simulink library "lib_fuel_converter"  (Simulink 4.00)
undefined symbols (not defined in the file): acc_mech_eff, acc_mech_pwr, acc_mech_trq, air_cp, amb_tmp, cyc_mph, ex_gas_cp, fc_acc_mass, fc_base_mass, fc_c2i_th_cond, fc_c_init_tmp, fc_cl2h_eff, fc_CO2_to_FUELgps, fc_cold, fc_cold_tmp, fc_cp, fc_ct_trq, fc_emisv, fc_ext_sarea, fc_fuel_den, fc_fuel_lhv, fc_h2x_th_cond, fc_h_air_flow, fc_h_cp, fc_h_init_tmp, fc_hood_emisv, fc_hood_sarea, fc_i2x_th_cond, fc_i_init_tmp, fc_inertia, fc_map_spd, fc_map_trq, fc_max_trq, fc_nn_model_name, fc_pwr_scale, fc_spd_scale, fc_trq_scale, fc_tstat, fc_x_init_tmp, fd_ratio, gb_num_init, gb_ratio, pow, vc_idle_spd, vc_key_on, veh_glider_mass, veh_mass, wh_radius
libraries: lib_fuel_converter x6, lib_etc x4
(part 1 of 4)
settings Model: Creator=NREL  LastModifiedBy=abrooker  ModifiedComment=abrooker -- Wed Jun 19 09:43:22 2002 -- Version 3.0440
settings Model: ModifiedHistory=|
  | abrooker -- Wed Jun 19 09:43:22 2002 -- Version 3.0440
  | 
  | 
  | abrooker -- Thu May 02 16:55:00 2002 -- Version 3.0439
  | deleted obsolete saber fc's
  | 
  | mokeefe -- Wed May 01 08:51:04 2002 -- Version 3.0438
  | changed the way scaling occurs on the FC temperature correction in the EO emissions and fuel usage block
  | 
  | tmarkel -- Tue Apr 30 08:52:52 2002 -- Version 3.0437
  | removed fuel cell model - moved to lib_fuel_cell
  | 
  | 
  | kharalds -- Thu Apr 25 16:04:02 2002 -- Version 3.0436
  | Removed the 4th input to Multi-port switches 1, 2, 3, 4 & blank (no number).
  | 
  | kharalds -- Fri Apr 19 16:04:21 2002 -- Version 3.0435
  | Removed fuel cell model option # 4 and its connections.
  | 
  | kharalds -- Fri Apr 19 08:05:59 2002 -- Version 3.0434
  | 
  | 
  | kharalds -- Fri Apr 19 08:04:37 2002 -- Version 3.0433
  | 
  | 
  | kharalds -- Thu Apr 18 18:08:33 2002 -- Version 3.0432
  | 
  | 
  | kharalds -- Thu Apr 18 18:05:53 2002 -- Version 3.0431
  | 
  | 
  | kharalds -- Thu Apr 18 18:00:41 2002 -- Version 3.0430
  | 
  | 
  | mokeefe -- Thu Apr 18 08:34:16 2002 -- Version 3.0429
  | saving the model:
  | o "without the model browser open"
  | o with only top-level screen visible
  | o with "fit to view" enabled
  | o with "status bar" off and "toolbar" off
  | o with "prompt to update model history with each save" on
  | 
  | kharalds -- Thu Apr 11 18:04:51 2002 -- Version 3.0250
  | changes in modified Springer fuel cell model/Fuel cell stack
  | 
  | 
  | kharalds -- Thu Apr 11 18:04:51 2002 -- Version 3.0250
  | changes in modified Springer fuel cell model/Fuel cell stack
  | 
  | 
  | kharalds -- Thu Apr 11 17:31:07 2002 -- Version 3.0249
  | changes in modified Springer fuel cell model block
  | 
  | kharalds -- Thu Apr 11 17:18:13 2002 -- Version 3.0248
  | 
  | 
  | kharalds -- Thu Apr 11 17:15:16 2002 -- Version 3.0247
  | 
  | 
  | kharalds -- Thu Apr 11 17:12:55 2002 -- Version 3.0246
  | added connections for fuel cell model option # 4 (multiport switches)
  | 
  | 
  | kharalds -- Thu Apr 11 17:10:53 2002 -- Version 3.0245
  | 04/11/02 added connections for modified Springer fuel cell model
  | 
  | kharalds -- Thu Apr 11 16:55:05 2002 -- Version 3.0244
  | 
  | 
  | mokeefe -- Wed Apr 10 13:00:58 2002 -- Version 3.0243
  | fixed broken links
  | 
  | mokeefe -- Wed Apr 10 11:52:00 2002 -- Version 3.0242
  | added display help for neural net models
  | 
  | mokeefe -- Wed Apr 10 11:33:37 2002 -- Version 3.0241
  | deleted a bad link in the neural network model
  | 
  | mokeefe -- Wed Apr 10 09:55:59 2002 -- Version 3.0240
  | 
  | 
  | mokeefe -- Wed Apr 10 09:55:48 2002 -- Version 3.0239
  | 
  | 
  | mokeefe -- Wed Apr 10 09:49:37 2002 -- Version 3.0238
  | 
  | 
  | mokeefe -- Wed Apr 10 09:47:28 2002 -- Version 3.0237
  | updated to add an O2 lookup table block that had gotten mis-linked in the original version.
  | 
  | mokeefe -- Wed Apr 10 09:33:36 2002 -- Version 3.0236
  | fixed broken links in the Saber * fuel converter files
  | 
  | mokeefe -- Wed Apr 10 09:30:23 2002 -- Version 3.0235
  | fixed the configurable subsystem name to not have a newline character
  | 
  | mokeefe -- Tue Apr 09 16:13:42 2002 -- Version 3.0234
  | 
  | 
  | mokeefe -- Tue Apr 09 16:12:25 2002 -- Version 3.0233
  | implementing configurable subsystems for the "fuel use and EO emis" block (to allow switch out with the West Virginia University Neural Network models)
  | 
  | kharalds -- Thu Apr 04 16:49:01 2002 -- Version 3.0232
  | Introduced a subsystem (copied from polarization fuel cell model), and a multiport switch. The proper connections are howevere not yet implemented!
  | 
  | kharalds -- Thu Apr 04 16:45:05 2002 -- Version 3.0231
  | 
  | 
  | kharalds -- Thu Apr 04 16:36:08 2002 -- Version 3.0230
  | Added fc_model constant # 4 and connections (for a new FC model) in fuel cell system block
  | Removed erroneous block notes under auxiliary blocks (polarization FC model)
  | 
  | mokeefe -- Wed Mar 06 08:05:16 2002 -- Version 3.0229
  | added the acc_mech_spd_est block to series fuel converter
  | 
  | mokeefe -- Tue Mar 05 15:37:33 2002 -- Version 3.0228
  | adding the fc_spd_est tag for fuel converter for series
  | 
  | mokeefe -- Tue Mar 05 15:27:34 2002 -- Version 3.0227
  | added global goto tag fc_spd_est to fuel converter <fc> for series
  | 
  | mokeefe -- Tue Mar 05 15:27:31 2002 -- Version 3.0226
  | 
  | 
  | mokeefe -- Tue Mar 05 15:26:09 2002 -- Version 3.0225
  | 
  | 
  | mokeefe -- Mon Mar 04 08:06:58 2002 -- Version 3.0224
  | 
  | 
  | mokeefe -- Mon Mar 04 08:04:43 2002 -- Version 3.0223
  | in fuel converter <fc>, engine torque, removed the switch block that cuts fc_trq_out_a to zero when the clutch state equals one. Engine torque must be passed out of the engine so that the auxiliary block can pick it up. The devices using "clutch_state" already kill the torque to zero between _in and _out properties anyway, so this appears to have been redundant.
  | 
  | mokeefe -- Thu Feb 28 08:25:30 2002 -- Version 3.0222
  | 
  | 
  | mokeefe -- Thu Feb 28 08:25:02 2002 -- Version 3.0221
  | 
  | 
  | mokeefe -- Wed Feb 27 14:08:59 2002 -- Version 3.0220
  | 
  | 
  | mokeefe -- Mon Feb 25 16:05:48 2002 -- Version 3.0219
  | 
  | 
  | mokeefe -- Mon Feb 25 16:04:45 2002 -- Version 3.0218
  | changed fuel converter <fc> for series to eliminate auxiliary loads inside the engine model (moving to the auxiliary library)
  | 
  | mokeefe -- Fri Feb 15 09:26:47 2002 -- Version 3.0217
  | changed the engine speed estimator and fc_spd_out_a back to original
  | 
  | mokeefe -- Fri Feb 15 07:18:44 2002 -- Version 3.0216
  | 
  | 
  | mokeefe -- Fri Feb 15 07:18:18 2002 -- Version 3.0215
  | changed the definition of fc_spd_out_a back to the original spd_command signal
  | 
  | mokeefe -- Thu Feb 14 17:06:09 2002 -- Version 3.0214
  | updated fuel converter <fc> with auxiliary loads tags: acc_mech_trq_est and acc_mech_trq
  | 
  | mokeefe -- Thu Feb 14 15:04:58 2002 -- Version 3.0213
  | added acc_mech_trq_est FROM tag from accessory block to the engine speed estimator
  | 
  | mokeefe -- Thu Feb 14 10:51:22 2002 -- Version 3.0212
  | 
  | 
  | mokeefe -- Thu Feb 14 08:43:33 2002 -- Version 3.0211
  | deleted unconnected block in lib_fuel_converter
  | 
  | mokeefe -- Thu Feb 14 08:14:24 2002 -- Version 3.0210
  | update the fuel converter <fc> with new library blocks for accessories
  | 
  | ssprik -- Fri Nov 02 16:24:16 2001 -- Version 3.0209
  | added fc_fuel_rate as a 'to workspace' variable
  | 
  | abrooker -- Tue Oct 09 16:22:51 2001 -- Version 3.0208
  | updated saber cosim S-fun demux signals (from Joe)
  | 
  | tmarkel -- Thu Sep 27 09:07:46 2001 -- Version 3.0207
  | applied map based temperature correction block fixes to fuel cell fuel converter - same as was done in ic engine fuel converter
  | 
  | abrooker -- Mon Sep 17 09:57:12 2001 -- Version 3.0206
  | 
  | 
  | tmarkel -- Fri Sep 14 16:12:10 2001 -- Version 3.0205
  | set normalized temperature saturation block limits to 0 to 1 from -1 to 0 and removed extraneous fuel and emissions constituent saturation limits
  | 
  | range is 0 to 1 so that we do not extrapolate outside of the known region
  | 
  | the secondary saturation blocks were removed because they were redundant with the temperature limit saturation block
  | 
  | Only applied to basic fuel converter for now but should be applicable to all fuel converter models.
  | 
  | tmarkel -- Fri Sep 14 15:48:49 2001 -- Version 3.0204
  | 
  | 
  | tmarkel -- Fri Sep 14 15:06:09 2001 -- Version 3.0203
  | 
  | 
  | tmarkel -- Fri Sep 14 14:55:14 2001 -- Version 3.0202
  | updated saturation on normalized temperature range in block map based temp correct in fuel use and emissions from -1 to 0 to 0 to 1
  | added manual switches around all saturation blocks for testing purposes.
  | 
  | 
  | abrooker -- Thu Jul 26 13:36:31 2001 -- Version 3.0201
  | Updated to add 14V Aux Loads to acc_elec_pwr
  | 
  | abrooker -- Thu Jul 26 10:42:44 2001 -- Version 3.0200
  | changed Aux Loads 14V lib submodel to be in Library: sub_lib_models file
  | 
  | abrooker -- Thu Jul 26 10:31:48 2001 -- Version 3.0199
  | changed 14V aux loads sub model to sub lib model
  | 
  | abrooker -- Tue Jul 24 12:52:12 2001 -- Version 3.0196
  | Made fix to 14V Aux Loads
  | 
  | abrooker -- Tue Jul 24 11:43:48 2001 -- Version 3.0195
  | 
  | 
  | abrooker -- Tue Jul 24 11:43:18 2001 -- Version 3.0194
  | made changes to 42 V Aux Loads :multiply by key on
  | 
  | abrooker -- Tue Jul 24 11:43:12 2001 -- Version 3.0193
  | 
  | 
  | abrooker -- Tue Jul 24 11:38:39 2001 -- Version 3.0192
  | 
  | 
  | abrooker -- Tue Jul 24 11:37:11 2001 -- Version 3.0191
  | made changes to Aux Loads 14V
  | 
  | abrooker -- Tue Jul 24 11:28:05 2001 -- Version 3.0190
  | Created sub-model from Aux Loads 14V
  | 
  | arajagop -- Mon Jul 23 17:14:36 2001 -- Version 3.0189
  | 
  | 
  | arajagop -- Mon Jul 23 17:12:34 2001 -- Version 3.0188
  | 
  | 
  | arajagop -- Mon Jul 23 17:12:09 2001 -- Version 3.0187
  | 
  | 
  | arajagop -- Mon Jul 23 17:09:52 2001 -- Version 3.0186
  | 
  | 
  | arajagop -- Mon Jul 23 17:02:25 2001 -- Version 3.0185
  | 
  | 
  | abrooker -- Mon Jul 23 14:15:51 2001 -- Version 3.0184
  | 
  | 
  | abrooker -- Mon Jul 23 14:00:39 2001 -- Version 3.0183
  | connected "starter" arrow
  | 
  | 
  | mokeefe -- Thu Jul 19 15:10:44 2001 -- Version 3.0182
  | modified fuel converter for fuel cell so that it will work in ADVISOR v 3.2. Values for O2 in g/s are passed through (dummy values of zero) to comply with the new emissions blocks
  | 
  | vjohnson -- Tue Jul 03 10:43:46 2001 -- Version 3.0156
  | 
  | 
  | mokeefe -- Fri Jun 29 15:12:06 2001 -- Version 3.0155
  | 
  | added sub-model collection and substituted veh_mass+veh_cargo_mass  for veh_mass
  | 
  | mokeefe -- Fri Jun 29 14:55:50 2001 -- Version 3.0154
  | 
  | 
  | mokeefe -- Fri Jun 29 09:01:29 2001 -- Version 3.0153
  | 
  | updating fuel converter Saver SV <fc> for veh_mass to veh_mass+veh_cargo_mass
  | 
  | 
  | mokeefe -- Fri Jun 29 08:51:40 2001 -- Version 3.0152
  | 
  | replacing engine inertia calculation that uses veh_mass with veh_mass+veh_cargo_mass in fuel converter Saber DV <fc>
  | 
  | mokeefe -- Fri Jun 29 08:38:48 2001 -- Version 3.0151
  | 
  | changing veh_mass to veh_mass plus veh_cargo_mass in fuel converter <fc> for Saber custom
  | 
  | vjohnson -- Thu May 24 09:57:06 2001 -- Version 3.052
  | 
  | 
  | vjohnson -- Tue Mar 20 09:14:38 2001 -- Version 3.051
  | 
  | 
  | mokeefe -- Tue Mar 13 11:04:59 2001 -- Version 3.050
  | changed colors of my changes back to black and white defaults
  | 
  | mokeefe -- Tue Mar 13 11:02:05 2001 -- Version 3.049
  | changes made to the fuel converter <fc> for series block diagram. Accessory load information was being logged to the workspace immediately after calculation. However, in the event that the engine is off, the accessory load info was still logged to the workspace. Because the energy usage figure in post-processing builds off of this accessory loads info, errors were occuring in the energy calculations.
  | 
  | The accessory loads information is now logged as a 0 W in the event that the engine is off.
  | 
  | vjohnson -- Tue Jan 30 17:54:01 2001 -- Version 3.05
  | 
  | 
  | vjohnson -- Tue Jan 30 17:52:10 2001 -- Version 3.04
  | 
  | 
  | abrooker -- Thu Jan 18 13:40:16 2001 -- Version 3.03
  | 
  | 
  | ssprik -- Wed Nov 01 16:23:01 2000 -- Version 3.02
  | ss & tm Changed the normalized temperature for fuel use and emissions
  |       temperature corrections
  | under fuel_converter/fuel use and EO emis/fc temp correct
  |       Changed lambda calculation from (fc_tstat-u)/75 to (fc_tstat-u)/(fc_tstat-20)
  |           where u is engine coolant temp and 20 is the ambient temp for which
  |           this temperature correction was calibrated.
  |       Changed the saturation immediately after it to go to a maximum of 1
  |           instead of infinity so as to not overpenalize for temperatures below 20 deg C..
  | 
  | 
  | ssprik -- Wed Nov 01 15:30:00 2000 -- Version 3.01
  | enabled comment dialogue to prompt the person saving the model to add comments.

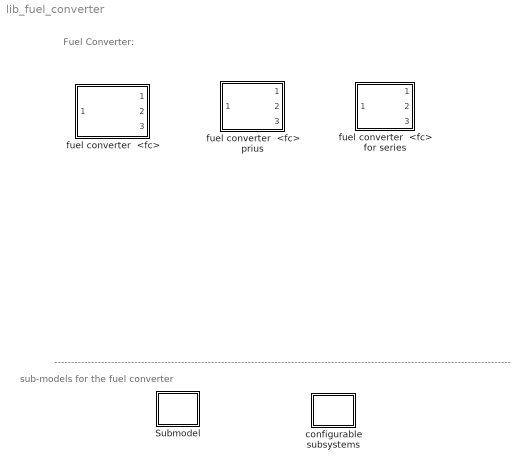
== system lib_fuel_converter ==
  note: Fuel Converter:
  note: -----------------------------------------------------------------------------------------------------------------------------------------
  note: sub-models
      | for the fuel converter
  Submodel : Subsystem
      settings: RTWFcnNameOpts=Auto  RTWFileNameOpts=Auto
  configurable subsystems : Subsystem
      settings: RTWFcnNameOpts=Auto  RTWFileNameOpts=Auto
  fuel converter  <fc> : Subsystem
      settings: RTWFcnNameOpts=Auto  RTWFileNameOpts=Auto
      mask Display: image(imread('bdi_fc.jpg'))
  fuel converter  <fc> for series : Subsystem
      settings: RTWFcnNameOpts=Auto  RTWFileNameOpts=Auto
      mask Display: image(imread('bdi_fc.jpg'))
  fuel converter  <fc> prius : Subsystem
      settings: RTWFcnNameOpts=Auto  RTWFileNameOpts=Auto
      mask Display: image(imread('bdi_fc.jpg'))

== system lib_fuel_converter/Submodel ==
  engine inertia as a function of total vehicle inertia (generous approximation) : Subsystem  Orientation=down
      settings: RTWFcnNameOpts=Auto  RTWFileNameOpts=Auto
  veh mass calc : Subsystem
      settings: RTWFcnNameOpts=Auto  RTWFileNameOpts=Auto

== system lib_fuel_converter/configurable subsystems ==
  fuel use and EO emis : Subsystem
      settings: RTWFcnNameOpts=Auto  RTWFileNameOpts=Auto
  fuel use and EO emis Configurable Subsystem : Subsystem  BlockChoice=fuel use and EO emis
      settings: TemplateBlock=self  MemberBlocks=fuel use and EO emis,fuel use and EO emis Neural Network Model  RTWFcnNameOpts=Auto  RTWFileNameOpts=Auto
  fuel use and EO emis Neural Network Model : Subsystem  mask{modelName=fc_nn_model_name}
      mask prompts: modelName "model no. (see help for specs)"
      mask help: Neural Network Model for Engine Fuel and Emissions Prediction
      mask init:
      | if strcmp(modelName,'1999CumminsISM370')
      |      modelNum=0;
      |      disp('Neural Net Model: 1999CumminsISM370')
      | elseif strcmp(modelName,'1994NavistarT444E')
      |      modelNum=1;
      |      disp('Neural Net Model: 1994NavistarT444E')
      | else
      |      modelNum=-1;
      |      disp('Neural Net Model: Invalid Setting!')
      |      disp('check value of fc_nn_model_name')
      | end
      settings: RTWFcnNameOpts=Auto  RTWFileNameOpts=Auto
      mask Help:
      | <h1>Neural Network Emissions Block Help</h1>
      | <h2>Introduction</h2>
      | <p>The neural network model takes engine shaft speed and torque and their time derivatives at 5 seconds and 10 seconds and predicts CO, CO2, and NOx emissions in g/s. Inputs to the model are speed (rpm) and torque (Nm). Outputs are CO, CO2, and NOx emissions in g/s.</p>
      | 
      | <p>There are neural network models trained for two engines thus far:</p>
      | <ol>
      | <li>1999 Cummins ISM 370</li>
      | <li>1994 Navistar T 444E</li>
      | </ol>
      | <p>In order to access the neural net models, one must type a string into the mask input screen. That string corresponds to:</p>
      | 
      | <table border=1>
      | <tr><td>Name</td><td>Engine</td></tr>
      | <tr><td>'1999CumminsISM370'</td><td>Cummins ISM 370</td></tr>
      | <tr><td>'1994NavistarT444E'</td><td>Navistar T 444E</td></tr>
      | </table>

== system lib_fuel_converter/fuel converter  <fc> ==
  torque and speed  req'd at engine  output shaft (Nm) : Inport  Port=1  LatchInput=off
  Block NOTES : Subsystem
      settings: RTWFcnNameOpts=Auto  RTWFileNameOpts=Auto
      mask Display: disp('Block\nNOTES')
  Demux : Demux  Outputs=2  BusSelectionMode=off
  Mux : Mux  Inputs=2
      settings: DisplayOption=none
  Mux1 : Mux  Inputs=2
      settings: DisplayOption=none
  To Workspace2 : ToWorkspace  VariableName=fc_trq_out_r  SampleTime=-1  SaveFormat=Array
  To Workspace3 : ToWorkspace  VariableName=fc_spd_out_r  SampleTime=-1  SaveFormat=Array
  To Workspace7 : ToWorkspace  VariableName=fc_brake_trq  SampleTime=-1  SaveFormat=Array
  To Workspace9 : ToWorkspace  VariableName=fc_spd_est  SampleTime=-1  SaveFormat=Array
  engine controller interface : Subsystem
      settings: RTWFcnNameOpts=Auto  RTWFileNameOpts=Auto
  engine speed estimator : Subsystem
      settings: RTWFcnNameOpts=Auto  RTWFileNameOpts=Auto
  engine torque : Subsystem
      settings: RTWFcnNameOpts=Auto  RTWFileNameOpts=Auto
  fuel use and EO emis Configurable Subsystem : Subsystem  BlockChoice=fuel use and EO emis
      settings: AttributesFormatString=%<BlockChoice>  TemplateBlock=lib_fuel_converter/configurable subsystems/fuel use and EO emis Configurable Subsystem  MemberBlocks=fuel use and EO emis,fuel use and EO emis Neural Network Model  RTWFcnNameOpts=Auto  RTWFileNameOpts=Auto
  help : Subsystem
      settings: OpenFcn=web(['file:\\\' which('fuel_converter.htm')]);  RTWFcnNameOpts=Auto  RTWFileNameOpts=Auto
      mask Display: image(imread('doc_man.jpg'))
  fuel use : Outport  Port=1  InitialOutput=0
  EO emis info : Outport  Port=2  InitialOutput=0
  "torque and speed  avail. to driveline (Nm), (rad/s)" : Outport  Port=3  InitialOutput=0
  tag scope: fc_brake_trq=global, fc_spd_est=global, fc_spd_out_a=global, fc_trq_out_a=global, fuel=global
  wires:
  engine torque/2(torque to shaft (Nm)) -> [fc_trq_out_a], Mux1/1
  engine torque/1(map torque (Nm)) -> fuel use and EO emis Configurable Subsystem/1(T (Nm)), To Workspace7/1, [fc_brake_trq]
  Mux1/1 -> "torque and speed  avail. to driveline (Nm), (rad/s)"/1
  fuel use and EO emis Configurable Subsystem/3(Vv,Tfc) -> Mux/2
  fuel use and EO emis Configurable Subsystem/2("FC ON?, EOem, MFex, Tex, O2ex") -> Mux/1
  Mux/1 -> EO emis info/1
  engine controller interface/1(spd command) -> engine torque/2(spd command), engine speed estimator/1(spd command), [fc_spd_out_a], Mux1/2
  Demux/1 -> engine torque/1(fc_trq_out_r), To Workspace2/1
  torque and speed  req'd at engine  output shaft (Nm)/1 -> Demux/1
  Demux/2 -> engine controller interface/1(fc_spd_out_r), To Workspace3/1, [fc_spd_out_r]
  fuel use and EO emis Configurable Subsystem/1(cumulative fuel  use (gal)) -> fuel use/1, [fuel]
  engine speed estimator/1(Out1) -> engine torque/3(engine spd), fuel use and EO emis Configurable Subsystem/2(w (rad/s)), To Workspace9/1, [fc_spd_est]

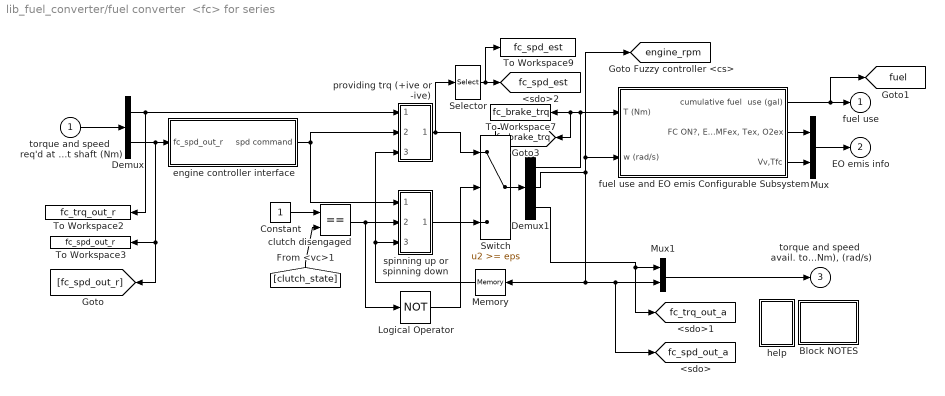
== system lib_fuel_converter/fuel converter  <fc> for series ==
  torque and speed  req'd at engine  output shaft (Nm) : Inport  Port=1  LatchInput=off
  Block NOTES : Subsystem
      settings: RTWFcnNameOpts=Auto  RTWFileNameOpts=Auto
      mask Display: disp('Block\nNOTES')
  Constant : Constant  Value=1
  Demux : Demux  Outputs=2  BusSelectionMode=off
  Demux1 : Demux  Outputs=3  BusSelectionMode=off
  Logical Operator : Logic  Operator=NOT  Inputs=1
  Memory : Memory  Orientation=left  X0=vc_idle_spd  InheritSampleTime=off
      settings: RTWStateStorageClass=Auto
  Mux : Mux  Inputs=2
      settings: DisplayOption=none
  Mux1 : Mux  Inputs=2
      settings: DisplayOption=none
  Selector : Selector  InputType=Vector  ElementSrc=Internal  Elements=[2]  RowSrc=Internal  Rows=1  ColumnSrc=Internal  Columns=1  InputPortWidth=3
  Switch : Switch  Threshold=eps
  To Workspace2 : ToWorkspace  VariableName=fc_trq_out_r  SampleTime=-1  SaveFormat=Array
  To Workspace3 : ToWorkspace  VariableName=fc_spd_out_r  SampleTime=-1  SaveFormat=Array
  To Workspace7 : ToWorkspace  VariableName=fc_brake_trq  SampleTime=-1  SaveFormat=Array
  To Workspace9 : ToWorkspace  VariableName=fc_spd_est  SampleTime=-1  SaveFormat=Array
  clutch disengaged : RelationalOperator  Operator===
  engine controller interface : Subsystem
      settings: RTWFcnNameOpts=Auto  RTWFileNameOpts=Auto
  fuel use and EO emis Configurable Subsystem : Subsystem  BlockChoice=fuel use and EO emis
      settings: AttributesFormatString=%<BlockChoice>  TemplateBlock=lib_fuel_converter/configurable subsystems/fuel use and EO emis Configurable Subsystem  MemberBlocks=fuel use and EO emis,fuel use and EO emis Neural Network Model  RTWFcnNameOpts=Auto  RTWFileNameOpts=Auto
  help : Subsystem
      settings: OpenFcn=web(['file:\\\' which('fuel_converter.htm')]);  RTWFcnNameOpts=Auto  RTWFileNameOpts=Auto
      mask Display: image(imread('doc_man.jpg'))
  providing trq (+ive or -ive) : Subsystem
      settings: RTWFcnNameOpts=Auto  RTWFileNameOpts=Auto
  spinning up or spinning down : Subsystem
      settings: RTWFcnNameOpts=Auto  RTWFileNameOpts=Auto
  fuel use : Outport  Port=1  InitialOutput=0
  EO emis info : Outport  Port=2  InitialOutput=0
  "torque and speed  avail. to driveline (Nm), (rad/s)" : Outport  Port=3  InitialOutput=0
  tag scope: engine_rpm=global, fc_brake_trq=global, fc_spd_est=global, fc_spd_out_a=global, fc_trq_out_a=global, fuel=global
  wires:
  Mux1/1 -> "torque and speed  avail. to driveline (Nm), (rad/s)"/1
  fuel use and EO emis Configurable Subsystem/3(Vv,Tfc) -> Mux/2
  fuel use and EO emis Configurable Subsystem/2("FC ON?, EOem, MFex, Tex, O2ex") -> Mux/1
  Mux/1 -> EO emis info/1
  Demux1/2 -> Mux1/2, [fc_spd_out_a], Memory/1, [engine_rpm], fuel use and EO emis Configurable Subsystem/2(w (rad/s))
  Demux1/3 -> Mux1/1, [fc_trq_out_a]
  Demux1/1 -> fuel use and EO emis Configurable Subsystem/1(T (Nm)), To Workspace7/1, [fc_brake_trq]
  engine controller interface/1(spd command) -> providing trq (+ive or -ive)/2(req'd spd (rad/s)), spinning up or spinning down/1(spd command (rad/s))
  torque and speed  req'd at engine  output shaft (Nm)/1 -> Demux/1
  Demux/1 -> To Workspace2/1, providing trq (+ive or -ive)/1(req'd trq (Nm))
  Demux/2 -> engine controller interface/1(fc_spd_out_r), To Workspace3/1, [fc_spd_out_r]
  clutch disengaged/1 -> spinning up or spinning down/2(engine disconnected from drivetrain), Logical Operator/1
  Constant/1 -> clutch disengaged/1
  [clutch_state] -> clutch disengaged/2
  Logical Operator/1 -> Switch/2
  providing trq (+ive or -ive)/1(map trq (Nm) spd (rad/s) trq to drivetrain (Nm)) -> Switch/1, Selector/1
  spinning up or spinning down/1(map trq (Nm) spd (rad/s) trq to drivetrain (Nm)) -> Switch/3
  Memory/1 -> spinning up or spinning down/3(previous engine spd (rad/s)), providing trq (+ive or -ive)/3(prev engine spd (rad/s))
  Switch/1 -> Demux1/1
  fuel use and EO emis Configurable Subsystem/1(cumulative fuel  use (gal)) -> fuel use/1, [fuel]
  Selector/1 -> [fc_spd_est], To Workspace9/1

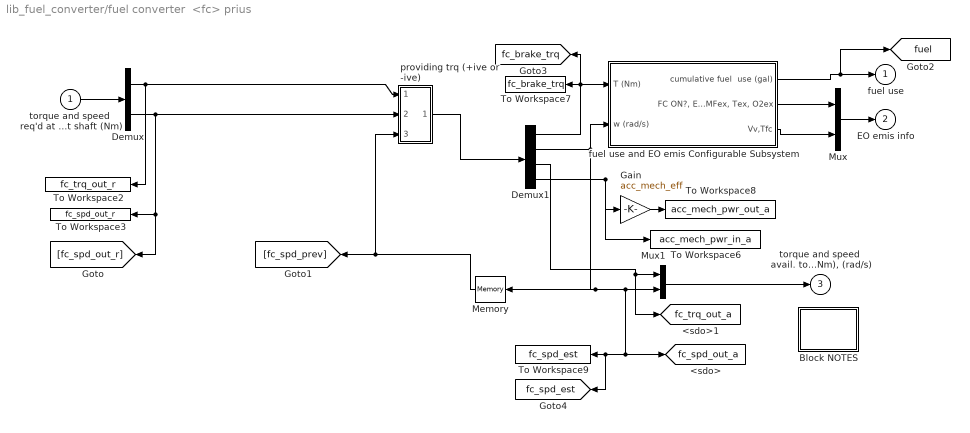
== system lib_fuel_converter/fuel converter  <fc> prius ==
  torque and speed  req'd at engine  output shaft (Nm) : Inport  Port=1  LatchInput=off
  Block NOTES : Subsystem
      settings: RTWFcnNameOpts=Auto  RTWFileNameOpts=Auto
      mask Display: disp('Block\nNOTES')
  Demux : Demux  Outputs=2  BusSelectionMode=off
  Demux1 : Demux  Outputs=4  BusSelectionMode=off
  Gain : Gain  Gain=acc_mech_eff  Multiplication=Element-wise(K.*u)  SaturateOnIntegerOverflow=on
  Memory : Memory  Orientation=left  X0=vc_idle_spd  InheritSampleTime=off
      settings: RTWStateStorageClass=Auto
  Mux : Mux  Inputs=2
      settings: DisplayOption=none
  Mux1 : Mux  Inputs=2
      settings: DisplayOption=none
  To Workspace2 : ToWorkspace  VariableName=fc_trq_out_r  SampleTime=-1  SaveFormat=Array
  To Workspace3 : ToWorkspace  VariableName=fc_spd_out_r  SampleTime=-1  SaveFormat=Array
  To Workspace6 : ToWorkspace  VariableName=acc_mech_pwr_in_a  SampleTime=-1  SaveFormat=Array
  To Workspace7 : ToWorkspace  VariableName=fc_brake_trq  SampleTime=-1  SaveFormat=Array
  To Workspace8 : ToWorkspace  VariableName=acc_mech_pwr_out_a  SampleTime=-1  SaveFormat=Array
  To Workspace9 : ToWorkspace  VariableName=fc_spd_est  SampleTime=-1  SaveFormat=Array
  fuel use and EO emis Configurable Subsystem : Subsystem  BlockChoice=fuel use and EO emis
      settings: AttributesFormatString=%<BlockChoice>  TemplateBlock=lib_fuel_converter/configurable subsystems/fuel use and EO emis Configurable Subsystem  MemberBlocks=fuel use and EO emis,fuel use and EO emis Neural Network Model  RTWFcnNameOpts=Auto  RTWFileNameOpts=Auto
  providing trq (+ive or -ive) : Subsystem
      settings: RTWFcnNameOpts=Auto  RTWFileNameOpts=Auto
  fuel use : Outport  Port=1  InitialOutput=0
  EO emis info : Outport  Port=2  InitialOutput=0
  "torque and speed  avail. to driveline (Nm), (rad/s)" : Outport  Port=3  InitialOutput=0
  tag scope: fc_brake_trq=global, fc_spd_est=global, fc_spd_out_a=global, fc_trq_out_a=global, fuel=global
  wires:
  Memory/1 -> [fc_spd_prev], providing trq (+ive or -ive)/3(prev engine spd (rad/s))
  providing trq (+ive or -ive)/1(map trq (Nm) spd (rad/s) trq to drivetrain (Nm) accessory load (W)) -> Demux1/1
  Demux/2 -> providing trq (+ive or -ive)/2(req'd spd (rad/s)), [fc_spd_out_r], To Workspace3/1
  Demux/1 -> providing trq (+ive or -ive)/1(req'd trq (Nm)), To Workspace2/1
  torque and speed  req'd at engine  output shaft (Nm)/1 -> Demux/1
  Demux1/1 -> fuel use and EO emis Configurable Subsystem/1(T (Nm)), To Workspace7/1, [fc_brake_trq]
  Demux1/3 -> [fc_trq_out_a], Mux1/1
  Demux1/2 -> Memory/1, [fc_spd_out_a], To Workspace9/1, [fc_spd_est], Mux1/2, fuel use and EO emis Configurable Subsystem/2(w (rad/s))
  Mux/1 -> EO emis info/1
  fuel use and EO emis Configurable Subsystem/2("FC ON?, EOem, MFex, Tex, O2ex") -> Mux/1
  fuel use and EO emis Configurable Subsystem/3(Vv,Tfc) -> Mux/2
  Gain/1 -> To Workspace8/1
  Demux1/4 -> Gain/1, To Workspace6/1
  Mux1/1 -> "torque and speed  avail. to driveline (Nm), (rad/s)"/1
  fuel use and EO emis Configurable Subsystem/1(cumulative fuel  use (gal)) -> fuel use/1, [fuel]

== system lib_fuel_converter/Submodel/engine inertia as a function of total vehicle inertia (generous approximation) ==
  Product : Product  Orientation=down  Inputs=*/  Multiplication=Element-wise(.*)  SaturateOnIntegerOverflow=on
  Sum : Sum  Orientation=down  Inputs=++|  SaturateOnIntegerOverflow=on
  engine inertia as a fraction of total vehicle inertia  (generous approximation)--denomenator : Fcn  Orientation=down  Expr=fc_inertia*(u*fd_ratio/wh_radius)^2
  engine inertia as a fraction of total vehicle inertia  (generous approximation)--numerator : Fcn  Orientation=down  Expr=fc_inertia*(u*fd_ratio/wh_radius)^2
  veh mass calc : lib_fuel_converter/Submodel/veh mass calc
      settings: RTWFcnNameOpts=Auto  RTWFileNameOpts=Auto
  Out1 : Outport  Orientation=down  Port=1
  wires:
  Product/1 -> Out1/1
  Sum/1 -> Product/2
  engine inertia as a fraction of total vehicle inertia  (generous approximation)--numerator/1 -> Product/1
  engine inertia as a fraction of total vehicle inertia  (generous approximation)--denomenator/1 -> Sum/2
  veh mass calc/1 -> Sum/1
  [gear_ratio] -> engine inertia as a fraction of total vehicle inertia  (generous approximation)--denomenator/1, engine inertia as a fraction of total vehicle inertia  (generous approximation)--numerator/1

== system lib_fuel_converter/Submodel/veh mass calc ==
  Constant : Constant  Value=veh_mass
  Sum : Sum  Inputs=|++  SaturateOnIntegerOverflow=on
  Out1 : Outport  Port=1
  wires:
  [veh_cargo_mass] -> Sum/1
  Constant/1 -> Sum/2
  Sum/1 -> Out1/1

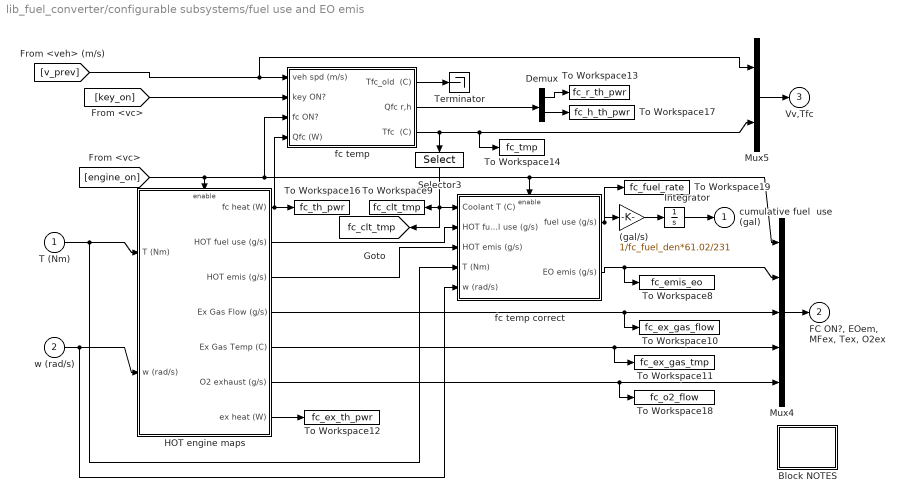
== system lib_fuel_converter/configurable subsystems/fuel use and EO emis ==
  T (Nm) : Inport  Port=1  LatchInput=off
  w (rad/s) : Inport  Port=2  LatchInput=off
  (gal/s) : Gain  Gain=1/fc_fuel_den*61.02/231  Multiplication=Element-wise(K.*u)  SaturateOnIntegerOverflow=on
  Block NOTES : Subsystem
      settings: RTWFcnNameOpts=Auto  RTWFileNameOpts=Auto
      mask Display: disp('Block\nNOTES')
  Demux : Demux  Outputs=2  BusSelectionMode=off
  "HOT engine maps " : Subsystem  TreatAsAtomicUnit=on
      settings: RTWFcnNameOpts=Auto  RTWFileNameOpts=Auto
  Integrator : Integrator  ExternalReset=none  InitialConditionSource=internal  InitialCondition=0  LimitOutput=off  UpperSaturationLimit=inf  LowerSaturationLimit=-inf  ShowSaturationPort=off  ShowStatePort=off  AbsoluteTolerance=auto
  Mux4 : Mux  Inputs=[1 4 1 1 1]
      settings: DisplayOption=none
  Mux5 : Mux  Inputs=[1 4 ]
      settings: DisplayOption=none
  Selector3 : Selector  Orientation=down  InputType=Vector  ElementSrc=Internal  Elements=2  RowSrc=Internal  Rows=1  ColumnSrc=Internal  Columns=1  InputPortWidth=4
  Terminator : Terminator
  To Workspace10 : ToWorkspace  VariableName=fc_ex_gas_flow  SampleTime=-1  SaveFormat=Array
  To Workspace11 : ToWorkspace  VariableName=fc_ex_gas_tmp  SampleTime=-1  SaveFormat=Array
  To Workspace12 : ToWorkspace  VariableName=fc_ex_th_pwr  SampleTime=-1  SaveFormat=Array
  To Workspace13 : ToWorkspace  VariableName=fc_r_th_pwr  SampleTime=-1  SaveFormat=Array
  To Workspace14 : ToWorkspace  VariableName=fc_tmp  SampleTime=-1  SaveFormat=Array
  To Workspace16 : ToWorkspace  VariableName=fc_th_pwr  SampleTime=-1  SaveFormat=Array
  To Workspace17 : ToWorkspace  VariableName=fc_h_th_pwr  SampleTime=-1  SaveFormat=Array
  To Workspace18 : ToWorkspace  VariableName=fc_o2_flow  SampleTime=-1  SaveFormat=Array
  To Workspace19 : ToWorkspace  VariableName=fc_fuel_rate  SampleTime=-1  SaveFormat=Array
  To Workspace8 : ToWorkspace  VariableName=fc_emis_eo  SampleTime=-1  SaveFormat=Array
  To Workspace9 : ToWorkspace  VariableName=fc_clt_tmp  SampleTime=-1  SaveFormat=Array
  fc temp : Subsystem
      settings: RTWFcnNameOpts=Auto  RTWFileNameOpts=Auto
  fc temp correct : Subsystem  TreatAsAtomicUnit=on
      settings: RTWFcnNameOpts=Auto  RTWFileNameOpts=Auto
  cumulative fuel  use (gal) : Outport  Port=1  InitialOutput=0
  "FC ON?, EOem, MFex, Tex, O2ex" : Outport  Port=2  InitialOutput=0
  Vv,Tfc : Outport  Port=3  InitialOutput=0
  tag scope: fc_clt_tmp=global
  wires:
  [key_on] -> fc temp/2(key ON?)
  [engine_on] -> "HOT engine maps "/Enable, fc temp/3(fc ON?), fc temp correct/Enable, Mux4/1
  fc temp correct/2(EO emis (g/s)) -> To Workspace8/1, Mux4/2
  Demux/2 -> To Workspace17/1
  Demux/1 -> To Workspace13/1
  fc temp/2(Qfc r,h) -> Demux/1
  "HOT engine maps "/1(fc heat (W)) -> To Workspace16/1, fc temp/4(Qfc (W))
  Selector3/1 -> fc temp correct/1(Coolant T (C)), To Workspace9/1, [fc_clt_tmp]
  "HOT engine maps "/7(ex heat (W)) -> To Workspace12/1
  fc temp/1(Tfc_old  (C)) -> Terminator/1
  fc temp/3(Tfc  (C)) -> Mux5/2, To Workspace14/1, Selector3/1
  "HOT engine maps "/3(HOT emis (g/s)) -> fc temp correct/3(HOT emis (g/s))
  "HOT engine maps "/2(HOT fuel use (g/s)) -> fc temp correct/2(HOT fuel use (g/s))
  (gal/s)/1 -> Integrator/1
  Integrator/1 -> cumulative fuel  use (gal)/1
  "HOT engine maps "/5(Ex Gas Temp (C)) -> To Workspace11/1, Mux4/4
  "HOT engine maps "/4(Ex Gas Flow (g/s)) -> To Workspace10/1, Mux4/3
  [v_prev] -> fc temp/1(veh spd (m/s)), Mux5/1
  Mux5/1 -> Vv,Tfc/1
  Mux4/1 -> "FC ON?, EOem, MFex, Tex, O2ex"/1
  w (rad/s)/1 -> "HOT engine maps "/2(w (rad/s)), fc temp correct/5(w (rad/s))
  T (Nm)/1 -> "HOT engine maps "/1(T (Nm)), fc temp correct/4(T (Nm))
  "HOT engine maps "/6(O2 exhaust (g/s)) -> Mux4/5, To Workspace18/1
  fc temp correct/1(fuel use (g/s)) -> (gal/s)/1, To Workspace19/1

== system lib_fuel_converter/configurable subsystems/fuel use and EO emis Configurable Subsystem ==
  T (Nm) : Inport  Port=1  LatchInput=off
  w (rad/s) : Inport  Port=2  LatchInput=off
  fuel use and EO emis : lib_fuel_converter/configurable subsystems/fuel use and EO emis
      settings: RTWFcnNameOpts=Auto  RTWFileNameOpts=Auto
  cumulative fuel  use (gal) : Outport  Port=1
  "FC ON?, EOem, MFex, Tex, O2ex" : Outport  Port=2
  Vv,Tfc : Outport  Port=3
  wires:
  T (Nm)/1 -> fuel use and EO emis/1
  w (rad/s)/1 -> fuel use and EO emis/2
  fuel use and EO emis/1 -> cumulative fuel  use (gal)/1
  fuel use and EO emis/2 -> "FC ON?, EOem, MFex, Tex, O2ex"/1
  fuel use and EO emis/3 -> Vv,Tfc/1

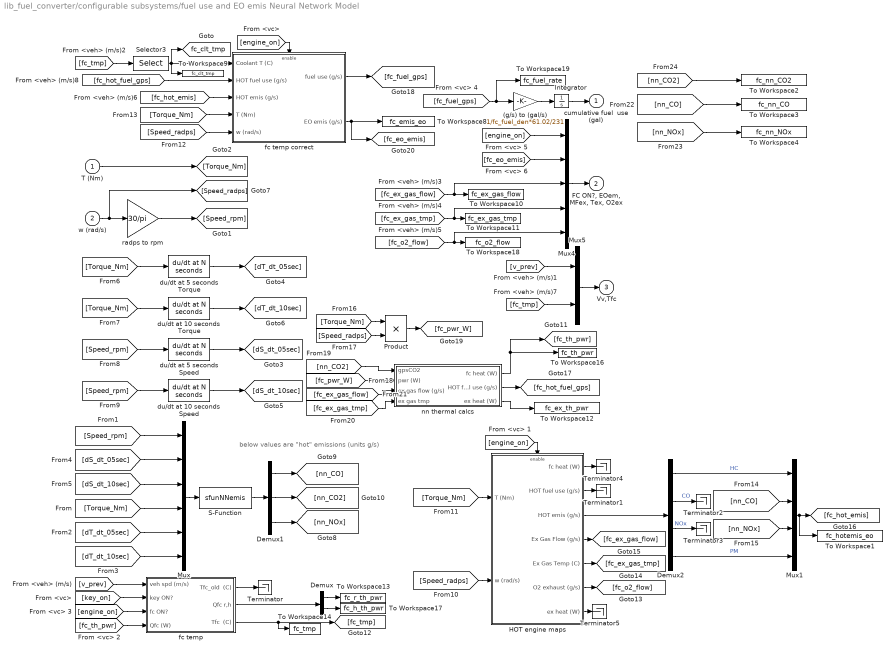
== system lib_fuel_converter/configurable subsystems/fuel use and EO emis Neural Network Model ==
  note: below values are "hot" emissions
      | (units g/s)
  T (Nm) : Inport  Port=1  LatchInput=off
  w (rad/s) : Inport  Port=2  LatchInput=off
  (g/s) to (gal/s) : Gain  Gain=1/fc_fuel_den*61.02/231  Multiplication=Element-wise(K.*u)  SaturateOnIntegerOverflow=on
  Demux : Demux  Outputs=2  BusSelectionMode=off
  Demux1 : Demux  Outputs=3  BusSelectionMode=off
  Demux2 : Demux  Outputs=4  BusSelectionMode=off
  "HOT engine maps " : Subsystem  TreatAsAtomicUnit=on
      settings: RTWFcnNameOpts=Auto  RTWFileNameOpts=Auto
  Integrator : Integrator  ExternalReset=none  InitialConditionSource=internal  InitialCondition=0  LimitOutput=off  UpperSaturationLimit=inf  LowerSaturationLimit=-inf  ShowSaturationPort=off  ShowStatePort=off  AbsoluteTolerance=auto
  Mux : Mux  Inputs=6
  Mux1 : Mux  Inputs=4
  Mux4 : Mux  Inputs=[1 4 1 1 1]
      settings: DisplayOption=none
  Mux5 : Mux  Inputs=[1 4 ]
      settings: DisplayOption=none
  Product : Product  Inputs=2  Multiplication=Element-wise(.*)  SaturateOnIntegerOverflow=on
  S-Function : S-Function  FunctionName=sfunNNemis  Parameters=modelNum  PortCounts=[]  SFunctionModules=''
  Selector3 : Selector  InputType=Vector  ElementSrc=Internal  Elements=2  RowSrc=Internal  Rows=1  ColumnSrc=Internal  Columns=1  InputPortWidth=4
  Terminator{,1..5} (6 alike) : Terminator
  To Workspace1 : ToWorkspace  VariableName=fc_hotemis_eo  SampleTime=-1  SaveFormat=Array
  To Workspace10 : ToWorkspace  VariableName=fc_ex_gas_flow  SampleTime=-1  SaveFormat=Array
  To Workspace11 : ToWorkspace  VariableName=fc_ex_gas_tmp  SampleTime=-1  SaveFormat=Array
  To Workspace12 : ToWorkspace  VariableName=fc_ex_th_pwr  SampleTime=-1  SaveFormat=Array
  To Workspace13 : ToWorkspace  VariableName=fc_r_th_pwr  SampleTime=-1  SaveFormat=Array
  To Workspace14 : ToWorkspace  VariableName=fc_tmp  SampleTime=-1  SaveFormat=Array
  To Workspace16 : ToWorkspace  VariableName=fc_th_pwr  SampleTime=-1  SaveFormat=Array
  To Workspace17 : ToWorkspace  VariableName=fc_h_th_pwr  SampleTime=-1  SaveFormat=Array
  To Workspace18 : ToWorkspace  VariableName=fc_o2_flow  SampleTime=-1  SaveFormat=Array
  To Workspace19 : ToWorkspace  VariableName=fc_fuel_rate  SampleTime=-1  SaveFormat=Array
  To Workspace2 : ToWorkspace  VariableName=fc_nn_CO2  SampleTime=-1  SaveFormat=Array
  To Workspace3 : ToWorkspace  VariableName=fc_nn_CO  SampleTime=-1  SaveFormat=Array
  To Workspace4 : ToWorkspace  VariableName=fc_nn_NOx  SampleTime=-1  SaveFormat=Array
  To Workspace8 : ToWorkspace  VariableName=fc_emis_eo  SampleTime=-1  SaveFormat=Array
  To Workspace9 : ToWorkspace  VariableName=fc_clt_tmp  SampleTime=-1  SaveFormat=Array
  du/dt at 10 seconds Speed : lib_etc/du//dt at N seconds  delay=10
  du/dt at 10 seconds Torque : lib_etc/du//dt at N seconds  delay=10
  du/dt at 5 seconds Speed : lib_etc/du//dt at N seconds  delay=5
  du/dt at 5 seconds Torque : lib_etc/du//dt at N seconds  delay=5
  fc temp : Subsystem
      settings: RTWFcnNameOpts=Auto  RTWFileNameOpts=Auto
  fc temp correct : Subsystem  TreatAsAtomicUnit=on
      settings: RTWFcnNameOpts=Auto  RTWFileNameOpts=Auto
  nn thermal calcs : Subsystem
      settings: RTWFcnNameOpts=Auto  RTWFileNameOpts=Auto
  radps to rpm : Gain  Gain=30/pi  Multiplication=Element-wise(K.*u)  SaturateOnIntegerOverflow=on
  cumulative fuel  use (gal) : Outport  Port=1  InitialOutput=0
  "FC ON?, EOem, MFex, Tex, O2ex" : Outport  Port=2  InitialOutput=0
  Vv,Tfc : Outport  Port=3  InitialOutput=0
  tag scope: fc_clt_tmp=global
  wires:
  [engine_on] -> fc temp correct/Enable
  fc temp correct/2(EO emis (g/s)) -> To Workspace8/1, [fc_eo_emis]
  Selector3/1 -> fc temp correct/1(Coolant T (C)), To Workspace9/1, [fc_clt_tmp]
  Mux5/1 -> Vv,Tfc/1
  w (rad/s)/1 -> radps to rpm/1, [Speed_radps]
  radps to rpm/1 -> [Speed_rpm]
  T (Nm)/1 -> [Torque_Nm]
  [Torque_Nm] -> du/dt at 5 seconds Torque/1
  [Torque_Nm] -> du/dt at 10 seconds Torque/1
  [Speed_rpm] -> du/dt at 5 seconds Speed/1
  [Speed_rpm] -> du/dt at 10 seconds Speed/1
  du/dt at 5 seconds Torque/1 -> [dT_dt_05sec]
  du/dt at 5 seconds Speed/1 -> [dS_dt_05sec]
  du/dt at 10 seconds Speed/1 -> [dS_dt_10sec]
  du/dt at 10 seconds Torque/1 -> [dT_dt_10sec]
  Mux/1 -> S-Function/1
  S-Function/1 -> Demux1/1
  Demux1/1 -> [nn_CO]
  Demux1/2 -> [nn_CO2]
  Demux1/3 -> [nn_NOx]
  [v_prev] -> Mux5/1
  [fc_tmp] -> Selector3/1
  [key_on] -> fc temp/2(key ON?)
  Demux/2 -> To Workspace17/1
  Demux/1 -> To Workspace13/1
  fc temp/2(Qfc r,h) -> Demux/1
  fc temp/1(Tfc_old  (C)) -> Terminator/1
  fc temp/3(Tfc  (C)) -> To Workspace14/1, [fc_tmp]
  [v_prev] -> fc temp/1(veh spd (m/s))
  [fc_th_pwr] -> fc temp/4(Qfc (W))
  [engine_on] -> fc temp/3(fc ON?)
  [fc_hot_emis] -> fc temp correct/3(HOT emis (g/s))
  "HOT engine maps "/5(Ex Gas Temp (C)) -> [fc_ex_gas_tmp]
  "HOT engine maps "/4(Ex Gas Flow (g/s)) -> [fc_ex_gas_flow]
  "HOT engine maps "/6(O2 exhaust (g/s)) -> [fc_o2_flow]
  [Torque_Nm] -> "HOT engine maps "/1(T (Nm))
  [Speed_radps] -> "HOT engine maps "/2(w (rad/s))
  [engine_on] -> "HOT engine maps "/Enable
  "HOT engine maps "/2(HOT fuel use (g/s)) -> Terminator1/1
  [fc_tmp] -> Mux5/2
  [fc_ex_gas_flow] -> To Workspace10/1, Mux4/3
  [fc_ex_gas_tmp] -> To Workspace11/1, Mux4/4
  [fc_o2_flow] -> To Workspace18/1, Mux4/5
  Mux4/1 -> "FC ON?, EOem, MFex, Tex, O2ex"/1
  [Speed_rpm] -> Mux/1
  [dS_dt_05sec] -> Mux/2
  [dS_dt_10sec] -> Mux/3
  [Torque_Nm] -> Mux/4
  [dT_dt_05sec] -> Mux/5
  [dT_dt_10sec] -> Mux/6
  [Torque_Nm] -> fc temp correct/4(T (Nm))
  [Speed_radps] -> fc temp correct/5(w (rad/s))
  Mux1/1 -> [fc_hot_emis], To Workspace1/1
  "HOT engine maps "/3(HOT emis (g/s)) -> Demux2/1
  Demux2/1 -> Mux1/1  "HC"
  Demux2/4 -> Mux1/4  "PM"
  Demux2/2 -> Terminator2/1  "CO"
  Demux2/3 -> Terminator3/1  "NOx"
  [nn_CO] -> Mux1/2
  [nn_NOx] -> Mux1/3
  "HOT engine maps "/1(fc heat (W)) -> Terminator4/1
  "HOT engine maps "/7(ex heat (W)) -> Terminator5/1
  nn thermal calcs/3(ex heat (W)) -> To Workspace12/1
  nn thermal calcs/1(fc heat (W)) -> [fc_th_pwr], To Workspace16/1
  nn thermal calcs/2(HOT fuel use (g/s)) -> [fc_hot_fuel_gps]
  [fc_hot_fuel_gps] -> fc temp correct/2(HOT fuel use (g/s))
  fc temp correct/1(fuel use (g/s)) -> [fc_fuel_gps]
  (g/s) to (gal/s)/1 -> Integrator/1
  Integrator/1 -> cumulative fuel  use (gal)/1
  [fc_fuel_gps] -> (g/s) to (gal/s)/1, To Workspace19/1
  [Torque_Nm] -> Product/1
  [Speed_radps] -> Product/2
  Product/1 -> [fc_pwr_W]
  [nn_CO2] -> nn thermal calcs/1(gpsCO2)
  [fc_pwr_W] -> nn thermal calcs/2(pwr (W))
  [fc_ex_gas_flow] -> nn thermal calcs/3(ex gas flow (g/s))
  [fc_ex_gas_tmp] -> nn thermal calcs/4(ex gas tmp)
  [engine_on] -> Mux4/1
  [fc_eo_emis] -> Mux4/2
  [nn_CO2] -> To Workspace2/1
  [nn_CO] -> To Workspace3/1
  [nn_NOx] -> To Workspace4/1

== system lib_fuel_converter/fuel converter  <fc>/Block NOTES ==
  note: This block models the internal combustion engine, and includes inertia effects,
      | performance limits, accessory loads, and temperature transient effects on fuel
      | use, engine-out emissions, and catalyst efficiency.  There are 'leads' to the
      | engine controller here, which controller determines whether the engine is on.

== system lib_fuel_converter/fuel converter  <fc>/engine controller interface ==
  fc_spd_out_r : Inport  Port=1  LatchInput=off
  spd command : Outport  Port=1
  tag scope: fc_spd_out_r=global
  wires:
  fc_spd_out_r/1 -> [fc_spd_out_r]
  [spd_command] -> spd command/1

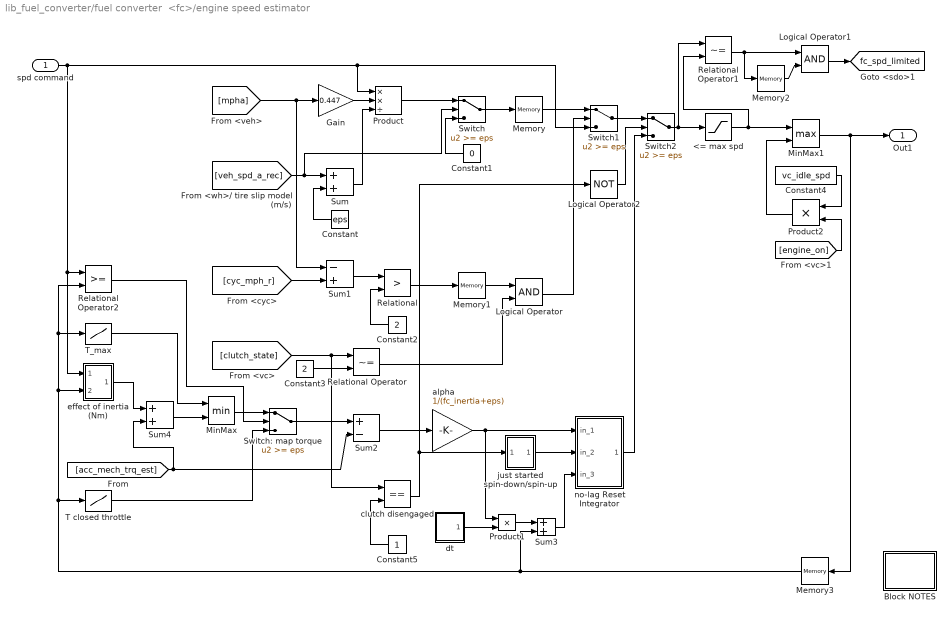
== system lib_fuel_converter/fuel converter  <fc>/engine speed estimator ==
  spd command : Inport  Port=1  LatchInput=off
  <= max spd : Saturate  UpperLimit=max(fc_map_spd)*fc_spd_scale  LowerLimit=-inf  LinearizeAsGain=on
  Block NOTES : Subsystem
      settings: RTWFcnNameOpts=Auto  RTWFileNameOpts=Auto
      mask Display: disp('Block\nNOTES')
  Constant : Constant  Orientation=left  Value=eps
  Constant1 : Constant  Orientation=left  Value=0
  Constant2 : Constant  Orientation=left  Value=2
  Constant3 : Constant  Value=2
  Constant4 : Constant  Value=vc_idle_spd
  Constant5 : Constant  Orientation=left  Value=1
  Gain : Gain  Gain=0.447  Multiplication=Element-wise(K.*u)  SaturateOnIntegerOverflow=on
  Logical Operator : Logic  Operator=AND  Inputs=2
  Logical Operator1 : Logic  Operator=AND  Inputs=2
  Logical Operator2 : Logic  Operator=NOT  Inputs=1
  Memory : Memory  X0=cyc_mph(1,2)*0.447/wh_radius*fd_ratio*gb_ratio(gb_num_init)  InheritSampleTime=off
      settings: RTWStateStorageClass=Auto
  Memory1 : Memory  X0=0  InheritSampleTime=off
      settings: RTWStateStorageClass=Auto
  Memory2 : Memory  X0=0  InheritSampleTime=off
      settings: RTWStateStorageClass=Auto
  Memory3 : Memory  Orientation=left  X0=cyc_mph(1,2)*0.447/wh_radius*fd_ratio*max(gb_ratio)  InheritSampleTime=off
      settings: RTWStateStorageClass=Auto
  MinMax : MinMax  Function=min  Inputs=2
  MinMax1 : MinMax  Function=max  Inputs=2
  Product : Product  Inputs=**/  Multiplication=Element-wise(.*)  SaturateOnIntegerOverflow=on
  Product1 : Product  Inputs=2  Multiplication=Element-wise(.*)  SaturateOnIntegerOverflow=on
  Product2 : Product  Orientation=left  Inputs=2  Multiplication=Element-wise(.*)  SaturateOnIntegerOverflow=on
  Relational : RelationalOperator  Operator=>
  Relational Operator : RelationalOperator  Operator=~=
  Relational Operator1 : RelationalOperator  Operator=~=
  Relational Operator2 : RelationalOperator  Operator=>=
  Sum : Sum  Inputs=++  SaturateOnIntegerOverflow=on
  Sum1 : Sum  Inputs=-+  SaturateOnIntegerOverflow=on
  Sum2 : Sum  Inputs=+-  SaturateOnIntegerOverflow=on
  Sum3 : Sum  Inputs=++  SaturateOnIntegerOverflow=on
  Sum4 : Sum  Inputs=++  SaturateOnIntegerOverflow=on
  Switch : Switch  Threshold=eps
  Switch1 : Switch  Threshold=eps
  Switch2 : Switch  Threshold=eps
  Switch: map torque : Switch  Threshold=eps
  T closed throttle : Lookup  InputValues=fc_map_spd*fc_spd_scale  OutputValues=fc_ct_trq*fc_trq_scale
  T_max : Lookup  InputValues=fc_map_spd*fc_spd_scale  OutputValues=fc_max_trq*fc_trq_scale
  alpha : Gain  Gain=1/(fc_inertia+eps)  Multiplication=Element-wise(K.*u)  SaturateOnIntegerOverflow=on
  clutch disengaged : RelationalOperator  Operator===
  dt : Subsystem
      settings: RTWFcnNameOpts=Auto  RTWFileNameOpts=Auto
  effect of inertia (Nm) : Subsystem
      settings: RTWFcnNameOpts=Auto  RTWFileNameOpts=Auto
  just started spin-down/spin-up : Subsystem
      settings: RTWFcnNameOpts=Auto  RTWFileNameOpts=Auto
  no-lag Reset Integrator : Subsystem  mask(No-lag Reset Integrator){@1=vc_idle_spd}
      mask prompts: @1 "Initial Value"
      mask help: No-lag Reset Integrator
      mask init:
      | initval=@1;
      settings: RTWFcnNameOpts=Auto  RTWFileNameOpts=Auto
      mask Help: Integrates first input using Euler technique.\nAt the time step that input 2 <> zero,\noutput is reset to input 3.
      mask Display: disp('1/s\nw/ reset\nno lag')
  Out1 : Outport  Port=1
  tag scope: fc_spd_limited=global
  wires:
  Sum3/1 -> no-lag Reset Integrator/3(in_3)
  just started spin-down/spin-up/1(trigger) -> no-lag Reset Integrator/2(in_2)
  no-lag Reset Integrator/1(out_1) -> Switch2/3
  Logical Operator/1 -> Switch1/2
  Logical Operator2/1 -> Switch2/2
  spd command/1 -> Product/1, Switch1/3, effect of inertia (Nm)/1(req'd spd (rad/s)), Relational Operator2/1
  effect of inertia (Nm)/1((Nm)) -> Sum4/1
  Sum4/1 -> MinMax/2
  T_max/1 -> MinMax/1
  MinMax/1 -> Switch: map torque/1
  T closed throttle/1 -> Switch: map torque/3
  Relational Operator2/1 -> Switch: map torque/2
  Switch: map torque/1 -> Sum2/1
  Relational Operator1/1 -> Memory2/1, Logical Operator1/1
  Logical Operator1/1 -> [fc_spd_limited]
  Memory2/1 -> Logical Operator1/2
  Switch2/1 -> Relational Operator1/1, <= max spd/1
  Product2/1 -> MinMax1/2
  MinMax1/1 -> Memory3/1, Out1/1
  Constant4/1 -> Product2/1
  [engine_on] -> Product2/2
  <= max spd/1 -> MinMax1/1, Relational Operator1/2
  Memory3/1 -> T closed throttle/1, effect of inertia (Nm)/2(prev spd), T_max/1, Relational Operator2/2, Sum3/2
  [clutch_state] -> clutch disengaged/1, Relational Operator/1
  clutch disengaged/1 -> just started spin-down/spin-up/1(state), Logical Operator2/1
  Switch1/1 -> Switch2/1
  Constant5/1 -> clutch disengaged/2
  alpha/1 -> no-lag Reset Integrator/1(in_1), Product1/1
  Product1/1 -> Sum3/1
  dt/1(out_1) -> Product1/2
  Sum2/1 -> alpha/1
  Constant3/1 -> Relational Operator/2
  Memory1/1 -> Logical Operator/1
  Relational Operator/1 -> Logical Operator/2
  Sum/1 -> Product/3
  Gain/1 -> Product/2
  Switch/1 -> Memory/1
  Relational/1 -> Memory1/1
  Sum1/1 -> Relational/1
  Constant2/1 -> Relational/2
  [mpha] -> Sum1/1, Gain/1
  [cyc_mph_r] -> Sum1/2
  Constant/1 -> Sum/2
  Memory/1 -> Switch1/1
  Constant1/1 -> Switch/3
  [veh_spd_a_rec] -> Switch/2, Sum/1
  Product/1 -> Switch/1
  [acc_mech_trq_est] -> Sum4/2, Sum2/2

== system lib_fuel_converter/fuel converter  <fc>/engine torque ==
  fc_trq_out_r : Inport  Port=1  LatchInput=off
  spd command : Inport  Port=2  LatchInput=off
  engine spd : Inport  Port=3  LatchInput=off
  Block NOTES : Subsystem
      settings: RTWFcnNameOpts=Auto  RTWFileNameOpts=Auto
      mask Display: disp('Block\nNOTES')
  Constant1 : Constant  Value=0
  Constant3 : Constant  Value=1
  Logical Operator : Logic  Operator=OR  Inputs=2
  MinMax : MinMax  Function=min  Inputs=2
  MinMax1 : MinMax  Function=max  Inputs=2
  Sum : Sum  Inputs=++  SaturateOnIntegerOverflow=on
  Sum1 : Sum  Inputs=+-  SaturateOnIntegerOverflow=on
  Switch : Switch  Threshold=eps
  Switch1 : Switch  Threshold=eps
  T_closed throttle : Subsystem
      settings: RTWFcnNameOpts=Auto  RTWFileNameOpts=Auto
  T_max : Subsystem
      settings: RTWFcnNameOpts=Auto  RTWFileNameOpts=Auto
  clutch not disengaged : RelationalOperator  Operator=~=
  effect of inertia (Nm) : Subsystem
      settings: RTWFcnNameOpts=Auto  RTWFileNameOpts=Auto
  engine commanded not to decelerate : RelationalOperator  Operator=<=
  limited : RelationalOperator  Operator=~=
  map torque (Nm) : Outport  Port=1
  torque to shaft (Nm) : Outport  Port=2
  tag scope: fc_trq_limited=global
  wires:
  spd command/1 -> engine commanded not to decelerate/2
  effect of inertia (Nm)/1((Nm)) -> Sum1/2, Sum/2
  fc_trq_out_r/1 -> Sum/1
  engine spd/1 -> effect of inertia (Nm)/1(engine spd (rad/s)), engine commanded not to decelerate/1, T_max/1(w_APU), T_closed throttle/1(w_APU)
  clutch not disengaged/1 -> Logical Operator/2, Switch1/2
  Switch/1 -> limited/1, MinMax/1
  MinMax1/1 -> Sum1/1, map torque (Nm)/1, limited/2
  T_closed throttle/1(T_closed throttle) -> MinMax1/2, Switch/3
  T_max/1(T_max) -> MinMax/2
  MinMax/1 -> MinMax1/1
  limited/1 -> [fc_trq_limited]
  Logical Operator/1 -> Switch/2
  Sum/1 -> Switch/1
  engine commanded not to decelerate/1 -> Logical Operator/1
  Constant3/1 -> clutch not disengaged/2
  [clutch_state] -> clutch not disengaged/1
  Switch1/1 -> torque to shaft (Nm)/1
  Sum1/1 -> Switch1/1
  Constant1/1 -> Switch1/3

== system lib_fuel_converter/fuel converter  <fc>/fuel use and EO emis Configurable Subsystem ==
  T (Nm) : Inport  Port=1  LatchInput=off
  w (rad/s) : Inport  Port=2  LatchInput=off
  fuel use and EO emis : lib_fuel_converter/configurable subsystems/fuel use and EO emis
      settings: RTWFcnNameOpts=Auto  RTWFileNameOpts=Auto
  cumulative fuel  use (gal) : Outport  Port=1
  "FC ON?, EOem, MFex, Tex, O2ex" : Outport  Port=2
  Vv,Tfc : Outport  Port=3
  wires:
  T (Nm)/1 -> fuel use and EO emis/1
  w (rad/s)/1 -> fuel use and EO emis/2
  fuel use and EO emis/1 -> cumulative fuel  use (gal)/1
  fuel use and EO emis/2 -> "FC ON?, EOem, MFex, Tex, O2ex"/1
  fuel use and EO emis/3 -> Vv,Tfc/1

== system lib_fuel_converter/fuel converter  <fc>/help ==

== system lib_fuel_converter/fuel converter  <fc> for series/Block NOTES ==
  note: This block models the internal combustion engine, and includes inertia effects,
      | performance limits, accessory loads, and temperature transient effects on fuel
      | use, engine-out emissions, and catalyst efficiency.  There are 'leads' to the
      | engine controller here, which controller determines whether the engine is on.

== system lib_fuel_converter/fuel converter  <fc> for series/engine controller interface ==
  fc_spd_out_r : Inport  Port=1  LatchInput=off
  spd command : Outport  Port=1
  tag scope: fc_spd_out_r=global
  wires:
  fc_spd_out_r/1 -> [fc_spd_out_r]
  [spd_command] -> spd command/1

== system lib_fuel_converter/fuel converter  <fc> for series/fuel use and EO emis Configurable Subsystem ==
  T (Nm) : Inport  Port=1  LatchInput=off
  w (rad/s) : Inport  Port=2  LatchInput=off
  fuel use and EO emis : lib_fuel_converter/configurable subsystems/fuel use and EO emis
      settings: RTWFcnNameOpts=Auto  RTWFileNameOpts=Auto
  cumulative fuel  use (gal) : Outport  Port=1
  "FC ON?, EOem, MFex, Tex, O2ex" : Outport  Port=2
  Vv,Tfc : Outport  Port=3
  wires:
  T (Nm)/1 -> fuel use and EO emis/1
  w (rad/s)/1 -> fuel use and EO emis/2
  fuel use and EO emis/1 -> cumulative fuel  use (gal)/1
  fuel use and EO emis/2 -> "FC ON?, EOem, MFex, Tex, O2ex"/1
  fuel use and EO emis/3 -> Vv,Tfc/1

== system lib_fuel_converter/fuel converter  <fc> for series/help ==
